simulink model "magball"  (Simulink 7.6)
settings: Solver=ode45  StartTime=0.0  StopTime=10  RelTol=1e-3
PreLoadFcn:
  | magballdat
  | magballop
values from neighbouring files (symbols this model uses):
  beta = 0.001    [magballdat.m]
  L = 0.02    [magballdat.m]    (also in scd_aero_guid_dat.m = 0.0065; scdaircraftpad.m = LinearAircraft.values(:,:,17); scdsaturationDFpad.m = zpk([],[0 -1 -10],1))
  m = 0.1    [magballdat.m]
  R = 2    [magballdat.m]    (also in scd_aero_guid_dat.m = 287.26; scdboilerpad.m = diag([1e2,1e6]); scddcmotorpad.m = [2,1.8,2.2])
libraries: simulink x1
settings Model: Creator=The MathWorks Inc.  BufferReuse=off
settings DataIOCC: InitialState=x0  SignalLoggingName=logsOut
settings OptimizationCC: BlockReduction=off  InlineParams=on  InlineInvariantSignals=on  BufferReuse=off  InitFltsAndDblsToZero=on
settings DebuggingCC: SaveWithParameterizedLinksMsg=none  SignalResolutionControl=TryResolveAllWithWarning  SolverPrmCheckMsg=none  MultiTaskDSMMsg=warning  StrictBusMsg=None
settings HardwareCC: TargetUnknown=on
settings CodeAppCC: CustomSymbolStrFcn=$F$N$M
settings GRTTargetCC: TargetFcnLib=ansi_tfl_tmw.mat

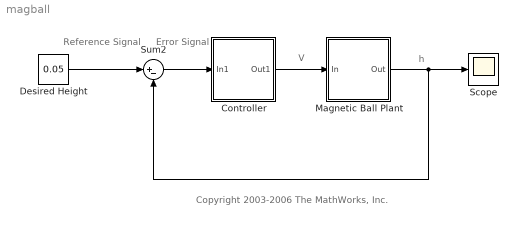
== system magball ==
  note: Error
      | Signal
  note: Reference
      | Signal
  note: V
  note: h
  note: Copyright 2003-2006 The MathWorks, Inc.
  Controller : Subsystem
      settings: RTWMemSecFuncInitTerm=Default  RTWMemSecFuncExecute=Default  RTWMemSecDataConstants=Default  RTWMemSecDataInternal=Default  RTWMemSecDataParameters=Default
  Desired Height : Constant  Value=0.05
  Magnetic Ball Plant : Subsystem
      settings: RTWMemSecFuncInitTerm=Default  RTWMemSecFuncExecute=Default  RTWMemSecDataConstants=Default  RTWMemSecDataInternal=Default  RTWMemSecDataParameters=Default
  Scope : Scope
  Sum2 : Sum  Inputs=|+-
  wires:
  Magnetic Ball Plant/1(Out) -> Scope/1, Sum2/2
  Sum2/1 -> Controller/1(In1)
  Controller/1(Out1) -> Magnetic Ball Plant/1(In)
  Desired Height/1 -> Sum2/1

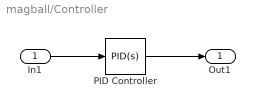
== system magball/Controller ==
  In1 : Inport
  PID Controller : simulink/Continuous/PID Controller  Tag=PID1  DialogController=pidpack.PIDConfig.pidDDGCreate  DialogControllerArgs=DataTag0  SystemSampleTime=-1  Controller=PID  TimeDomain=Continuous-time  SampleTime=1  IntegratorMethod=Forward Euler  FilterMethod=Forward Euler  Form=Parallel  P=-448.852140  I=-236.261487  D=-69.987148  N=995.837207  InitialConditionSource=internal  InitialConditionForIntegrator=14.0071  InitialConditionForFilter=0  ExternalReset=none  ZeroCross=off  LimitOutput=off  UpperSaturationLimit=inf  LowerSaturationLimit=-inf  LinearizeAsGain=off  AntiWindupMode=none  Kb=1  TrackingMode=off  Kt=1  PParamMin=[ ]  PParamMax=[ ]  IParamMin=[ ]  IParamMax=[ ]  DParamMin=[ ]  DParamMax=[ ]  NParamMin=[ ]  NParamMax=[ ]  KbParamMin=[ ]  KbParamMax=[ ]  KtParamMin=[ ]  KtParamMax=[ ]  POutMin=[ ]  POutMax=[ ]  IOutMin=[ ]  IOutMax=[ ]  DOutMin=[ ]  DOutMax=[ ]  NOutMin=[ ]  NOutMax=[ ]  KbOutMin=[ ]  KbOutMax=[ ]  KtOutMin=[ ]  KtOutMax=[ ]  IntegratorOutMin=[ ]  IntegratorOutMax=[ ]  FilterOutMin=[ ]  FilterOutMax=[ ]  SumOutMin=[ ]  SumOutMax=[ ]  SumI1OutMin=[ ]  SumI1OutMax=[ ]  SumI2OutMin=[ ]  SumI2OutMax=[ ]  SumI3OutMin=[ ]  SumI3OutMax=[ ]  SumDOutMin=[ ]  SumDOutMax=[ ]  SaturationOutMin=[ ]  SaturationOutMax=[ ]  IntegratorContinuousStateAttributes=''  IntegratorStateMustResolveToSignalObject=off  IntegratorRTWStateStorageClass=Auto  FilterContinuousStateAttributes=''  FilterStateMustResolveToSignalObject=off  FilterRTWStateStorageClass=Auto
  Out1 : Outport
  wires:
  In1/1 -> PID Controller/1
  PID Controller/1 -> Out1/1

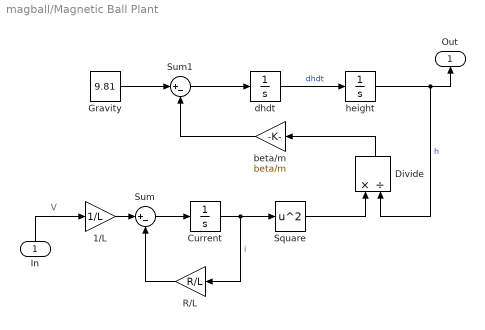
== system magball/Magnetic Ball Plant ==
  note: V
  In : Inport
  1/L : Gain  Gain=1/L
  Current : Integrator  InitialCondition=7.0036
  Divide : Product  Inputs=*/
  Gravity : Constant  Value=9.81
  R/L : Gain  Gain=R/L
  Square : Math  Operator=square  SaturateOnIntegerOverflow=on
  Sum : Sum  Inputs=|+-
  Sum1 : Sum  Inputs=|+-
  beta/m : Gain  Gain=beta/m
  dhdt : Integrator
  height : Integrator  InitialCondition=0.05
  Out : Outport
  wires:
  dhdt/1 -> height/1  "dhdt"
  height/1 -> Out/1, Divide/2  "h"
  Sum/1 -> Current/1
  1/L/1 -> Sum/1
  R/L/1 -> Sum/2
  Current/1 -> Square/1, R/L/1  "i"
  Square/1 -> Divide/1
  Divide/1 -> beta/m/1
  Gravity/1 -> Sum1/1
  beta/m/1 -> Sum1/2
  Sum1/1 -> dhdt/1
  In/1 -> 1/L/1
